simulink model "sim_Exp81_part4"  (R2019a)
settings: Solver=VariableStepAuto  StartTime=0.0  StopTime=10.0  RelTol=1e-3
undefined symbols (not defined in the file): GP_den, GP_num, Kp_part1, L, T
settings Model: Creator=sgxgong4  LastModifiedBy=sgxgong4

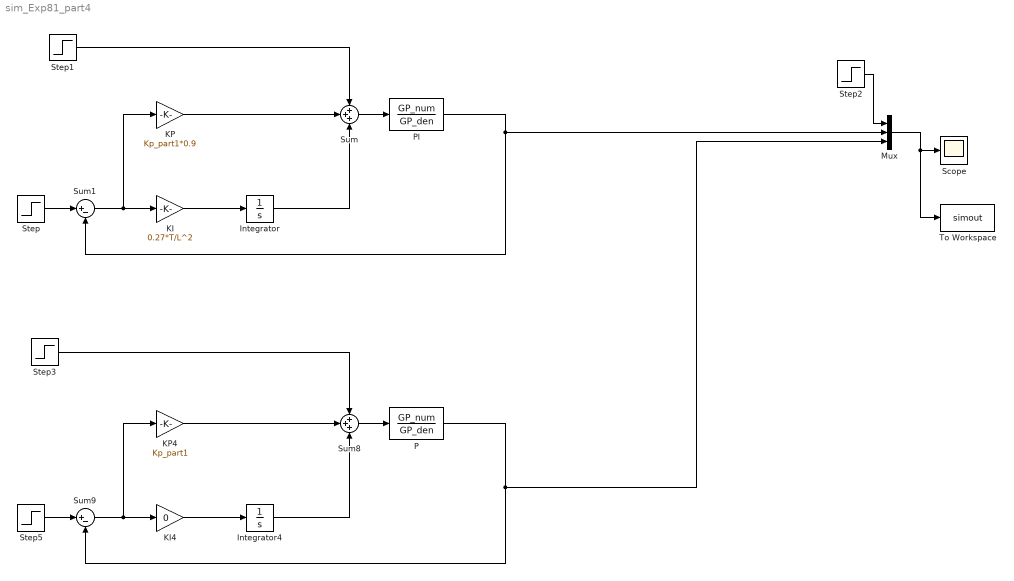
== system sim_Exp81_part4 ==
  Integrator : Integrator
  Integrator4 : Integrator
  KI : Gain  Gain=0.27*T/L^2
  KI4 : Gain  Gain=0
  KP : Gain  Gain=Kp_part1*0.9
  KP4 : Gain  Gain=Kp_part1
  Mux : Mux  Inputs=3
  P : TransferFcn  Numerator=GP_num  Denominator=GP_den
  PI : TransferFcn  Numerator=GP_num  Denominator=GP_den
  Scope : Scope
  Step : Step  Time=0  SampleTime=0
  Step1 : Step  Time=0  After=10  SampleTime=0
  Step2 : Step  Time=0  SampleTime=0
  Step3 : Step  Time=0  After=10  SampleTime=0
  Step5 : Step  Time=0  SampleTime=0
  Sum : Sum  Inputs=+++
  Sum1 : Sum  Inputs=|+-
  Sum8 : Sum  Inputs=+++
  Sum9 : Sum  Inputs=|+-
  To Workspace : ToWorkspace  VariableName=simout  SaveFormat=Structure With Time  SampleTime=-1
  wires:
  KI/1 -> Integrator/1
  KP/1 -> Sum/2
  Integrator/1 -> Sum/3
  Sum1/1 -> KP/1, KI/1
  Step/1 -> Sum1/1
  Sum/1 -> PI/1
  PI/1 -> Sum1/2, Mux/2
  Integrator4/1 -> Sum8/3
  Sum8/1 -> P/1
  Step5/1 -> Sum9/1
  Sum9/1 -> KP4/1, KI4/1
  KI4/1 -> Integrator4/1
  KP4/1 -> Sum8/2
  Step1/1 -> Sum/1
  Step2/1 -> Mux/1
  Mux/1 -> To Workspace/1, Scope/1
  Step3/1 -> Sum8/1
  P/1 -> Mux/3, Sum9/2
